simulink library "FUSA_EM_EMFR"  (R2023b)
settings: Solver=VariableStepAuto  StartTime=0.0  StopTime=10.0  RelTol=1e-3
undefined symbols (not defined in the file): FUSA_EM_EMFR_p1_TempMotDertCoefFrRi_na, FUSA_EM_EMFR_px_TempMotFrRiLkp_degC
libraries: simulink x1
settings Model: Creator=blatak  LastModifiedBy=blatak

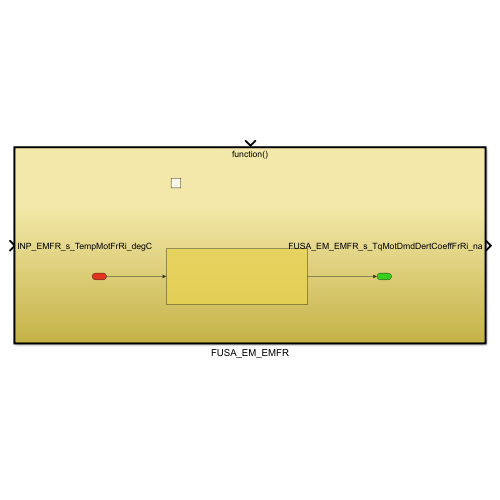
[thumbnail: Simulink's stored preview of the top-level diagram]
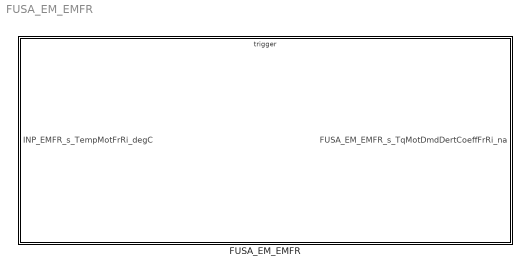
== system FUSA_EM_EMFR ==
  FUSA_EM_EMFR : Subsystem  TreatAsAtomicUnit=on

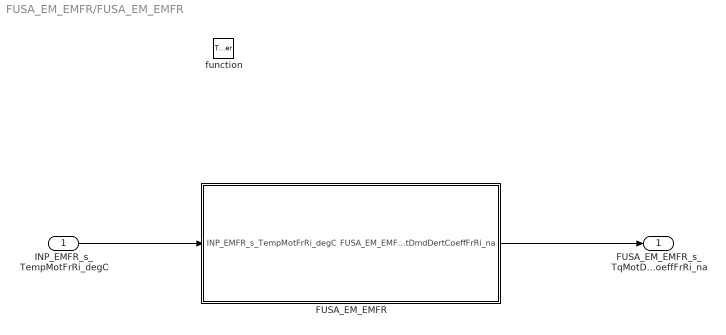
== system FUSA_EM_EMFR/FUSA_EM_EMFR ==
  INP_EMFR_s_TempMotFrRi_degC : Inport
  function : TriggerPort  TriggerType=function-call  VariantControl=(inherit)
  FUSA_EM_EMFR : Subsystem
  FUSA_EM_EMFR_s_TqMotDmdDertCoeffFrRi_na : Outport  Description=Derate torque coefficient front
  wires:
  INP_EMFR_s_TempMotFrRi_degC/1 -> FUSA_EM_EMFR/1(INP_EMFR_s_TempMotFrRi_degC)
  FUSA_EM_EMFR/1(FUSA_EM_EMFR_s_TqMotDmdDertCoeffFrRi_na) -> FUSA_EM_EMFR_s_TqMotDmdDertCoeffFrRi_na/1

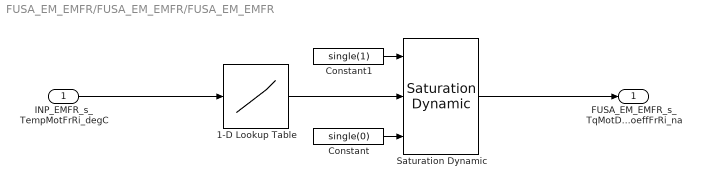
== system FUSA_EM_EMFR/FUSA_EM_EMFR/FUSA_EM_EMFR ==
  INP_EMFR_s_TempMotFrRi_degC : Inport
  1-D Lookup Table : Lookup_n-D  NumberOfTableDimensions=1  BreakpointsForDimension1=FUSA_EM_EMFR_px_TempMotFrRiLkp_degC  Table=FUSA_EM_EMFR_p1_TempMotDertCoefFrRi_na  InternalRulePriority=Speed  RndMeth=Simplest
  Constant : Constant  Value=single(0)
  Constant1 : Constant  Value=single(1)
  Saturation Dynamic : simulink/Discontinuities/Saturation Dynamic  OutMin=[]  OutMax=[]  OutDataTypeStr=Inherit: Same as second input  OutDataType=fixdt(1, 16)  OutScaling=2^-10  DoSatur=off
  FUSA_EM_EMFR_s_TqMotDmdDertCoeffFrRi_na : Outport  Description=Derate torque coefficient front
  wires:
  1-D Lookup Table/1 -> Saturation Dynamic/2
  Constant/1 -> Saturation Dynamic/3
  INP_EMFR_s_TempMotFrRi_degC/1 -> 1-D Lookup Table/1
  Constant1/1 -> Saturation Dynamic/1
  Saturation Dynamic/1 -> FUSA_EM_EMFR_s_TqMotDmdDertCoeffFrRi_na/1
